simulink model "ActiveComponents"  (Simulink 8.3)
settings: Solver=ode45  StartTime=0.0  StopTime=10.0  MaxStep=0.1  RelTol=1e-3
settings Model: Creator=Administrator  LastModifiedBy=Administrator
settings DataIOCC: SignalLoggingSaveFormat=Dataset
settings DebuggingCC: UnderspecifiedInitializationDetection=Simplified  StateNameClashWarn=none
settings GRTTargetCC: CombineOutputUpdateFcns=on  GRTInterface=off

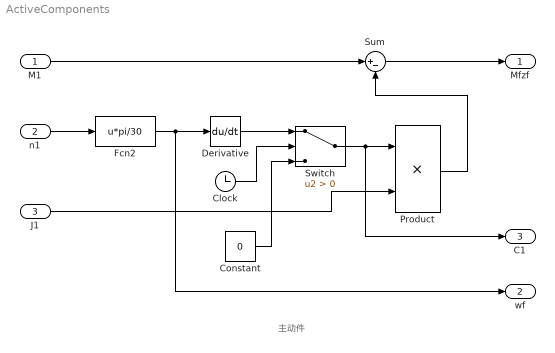
== system ActiveComponents ==
  note: 主动件
  M1 : Inport
  n1 : Inport  Port=2
  J1 : Inport  Port=3
  Clock : Clock
  Constant : Constant  Value=0
  Derivative : Derivative
  Fcn2 : Fcn  Expr=u*pi/30
  Product : Product
  Sum : Sum  Inputs=|+-
  Switch : Switch  Criteria=u2 > Threshold
  Mfzf : Outport
  wf : Outport  Port=2
  C1 : Outport  Port=3
  wires:
  n1/1 -> Fcn2/1
  Fcn2/1 -> wf/1, Derivative/1
  M1/1 -> Sum/1
  Derivative/1 -> Switch/1
  Clock/1 -> Switch/2
  J1/1 -> Product/2
  Switch/1 -> C1/1, Product/1
  Constant/1 -> Switch/3
  Product/1 -> Sum/2
  Sum/1 -> Mfzf/1
